simulink model "stream_mdbrt_backup5"  (R2023b)
settings: Solver=VariableStepAuto  StartTime=0.0  StopTime=(48)/fs  RelTol=1e-3
PreLoadFcn:
  | clear all;
  | 
  | fs = 100e6;
PostLoadFcn:
  | ratio = 1/6;
  | set(0,'units','pixels');
  | pixels = get(0,'screensize');
  | point1 = round(pixels(3)*ratio);
  | point2 = round(pixels(4)*ratio);
  | point3 = pixels(3)-round(pixels(3)*ratio);
  | point4 = pixels(4)-round(pixels(4)*ratio);
  | h = get_param(gcs,'handle');
  | set_param(h,'location',[point1 point2 point3 point4]);
  | pause(0.2);
  | set_param(h,'Zoomfactor','fit to view');
  | 
  | clear ratio pixels point1 point2 point3 point4 h
  | 
  | % https://uk.mathworks.com/matlabcentral/answers/358413-open-simulink-model-with-set-window-size-and-position
undefined symbols (not defined in the file): AXI4, bits, bitsheight, bitsiter, bitswidth, Lite, xc7z020clg400
libraries: hdlBasic x527, vmcUtilities x1
(part 5 of 5)

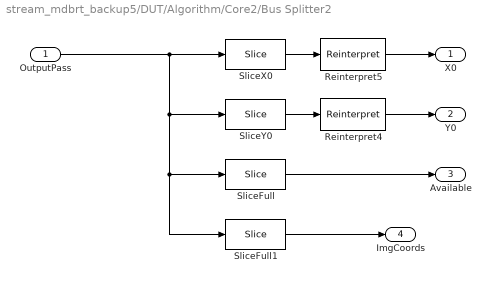
== system stream_mdbrt_backup5/DUT/Algorithm/Core2/Bus Splitter2 ==
  OutputPass : Inport
  Reinterpret4 : hdlBasic/Reinterpret  force_arith_type=on  arith_type="Signed  (2's comp)"  force_bin_pt=on  bin_pt=binpoint  XmcBlockStatus=1  maskContainerNames=group1  block_type=reinterpret  block_config=sysgen:Reinterpret_config
  Reinterpret5 : hdlBasic/Reinterpret  force_arith_type=on  arith_type="Signed  (2's comp)"  force_bin_pt=on  bin_pt=binpoint  XmcBlockStatus=1  maskContainerNames=group1  block_type=reinterpret  block_config=sysgen:Reinterpret_config
  SliceFull : hdlBasic/Slice  nbits=1  boolean_output=on  mode=Upper Bit Location + Width  bit1=0  base1=MSB of Input  bit0=0  base0=LSB of Input  XmcBlockStatus=1  maskContainerNames=group1  block_type=slice  block_config=sysgen:Slice_config
  SliceFull1 : hdlBasic/Slice  nbits=bitswidth+bitsheight  boolean_output=off  mode=Lower Bit Location + Width  bit1=0  base1=MSB of Input  bit0=0  base0=LSB of Input  XmcBlockStatus=1  maskContainerNames=group1  block_type=slice  block_config=sysgen:Slice_config
  SliceX0 : hdlBasic/Slice  nbits=bits  boolean_output=off  mode=Upper Bit Location + Width  bit1=-1-bits  base1=MSB of Input  bit0=0  base0=LSB of Input  XmcBlockStatus=1  maskContainerNames=group1  block_type=slice  block_config=sysgen:Slice_config
  SliceY0 : hdlBasic/Slice  nbits=bits  boolean_output=off  mode=Upper Bit Location + Width  bit1=-1  base1=MSB of Input  bit0=0  base0=LSB of Input  XmcBlockStatus=1  maskContainerNames=group1  block_type=slice  block_config=sysgen:Slice_config
  X0 : Outport
  Y0 : Outport  Port=2
  Available : Outport  Port=3
  ImgCoords : Outport  Port=4
  wires:
  Reinterpret5/1 -> X0/1
  SliceFull/1 -> Available/1
  Reinterpret4/1 -> Y0/1
  SliceX0/1 -> Reinterpret5/1
  SliceY0/1 -> Reinterpret4/1
  SliceFull1/1 -> ImgCoords/1
  OutputPass/1 -> SliceX0/1, SliceY0/1, SliceFull/1, SliceFull1/1

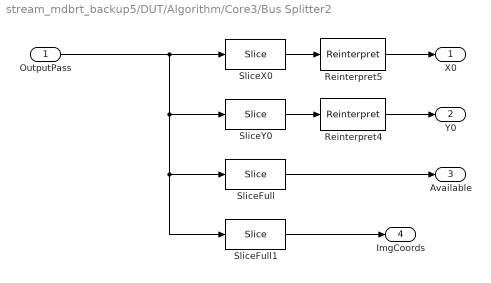
== system stream_mdbrt_backup5/DUT/Algorithm/Core3/Bus Splitter2 ==
  OutputPass : Inport
  Reinterpret4 : hdlBasic/Reinterpret  force_arith_type=on  arith_type="Signed  (2's comp)"  force_bin_pt=on  bin_pt=binpoint  XmcBlockStatus=1  maskContainerNames=group1  block_type=reinterpret  block_config=sysgen:Reinterpret_config
  Reinterpret5 : hdlBasic/Reinterpret  force_arith_type=on  arith_type="Signed  (2's comp)"  force_bin_pt=on  bin_pt=binpoint  XmcBlockStatus=1  maskContainerNames=group1  block_type=reinterpret  block_config=sysgen:Reinterpret_config
  SliceFull : hdlBasic/Slice  nbits=1  boolean_output=on  mode=Upper Bit Location + Width  bit1=0  base1=MSB of Input  bit0=0  base0=LSB of Input  XmcBlockStatus=1  maskContainerNames=group1  block_type=slice  block_config=sysgen:Slice_config
  SliceFull1 : hdlBasic/Slice  nbits=bitswidth+bitsheight  boolean_output=off  mode=Lower Bit Location + Width  bit1=0  base1=MSB of Input  bit0=0  base0=LSB of Input  XmcBlockStatus=1  maskContainerNames=group1  block_type=slice  block_config=sysgen:Slice_config
  SliceX0 : hdlBasic/Slice  nbits=bits  boolean_output=off  mode=Upper Bit Location + Width  bit1=-1-bits  base1=MSB of Input  bit0=0  base0=LSB of Input  XmcBlockStatus=1  maskContainerNames=group1  block_type=slice  block_config=sysgen:Slice_config
  SliceY0 : hdlBasic/Slice  nbits=bits  boolean_output=off  mode=Upper Bit Location + Width  bit1=-1  base1=MSB of Input  bit0=0  base0=LSB of Input  XmcBlockStatus=1  maskContainerNames=group1  block_type=slice  block_config=sysgen:Slice_config
  X0 : Outport
  Y0 : Outport  Port=2
  Available : Outport  Port=3
  ImgCoords : Outport  Port=4
  wires:
  OutputPass/1 -> SliceFull1/1, SliceFull/1, SliceY0/1, SliceX0/1
  SliceFull1/1 -> ImgCoords/1
  SliceY0/1 -> Reinterpret4/1
  SliceX0/1 -> Reinterpret5/1
  Reinterpret4/1 -> Y0/1
  SliceFull/1 -> Available/1
  Reinterpret5/1 -> X0/1

== system stream_mdbrt_backup5/DUT/Algorithm/Core4/Bus Splitter2 ==
  OutputPass : Inport
  Reinterpret4 : hdlBasic/Reinterpret  force_arith_type=on  arith_type="Signed  (2's comp)"  force_bin_pt=on  bin_pt=binpoint  XmcBlockStatus=1  maskContainerNames=group1  block_type=reinterpret  block_config=sysgen:Reinterpret_config
  Reinterpret5 : hdlBasic/Reinterpret  force_arith_type=on  arith_type="Signed  (2's comp)"  force_bin_pt=on  bin_pt=binpoint  XmcBlockStatus=1  maskContainerNames=group1  block_type=reinterpret  block_config=sysgen:Reinterpret_config
  SliceFull : hdlBasic/Slice  nbits=1  boolean_output=on  mode=Upper Bit Location + Width  bit1=0  base1=MSB of Input  bit0=0  base0=LSB of Input  XmcBlockStatus=1  maskContainerNames=group1  block_type=slice  block_config=sysgen:Slice_config
  SliceFull1 : hdlBasic/Slice  nbits=bitswidth+bitsheight  boolean_output=off  mode=Lower Bit Location + Width  bit1=0  base1=MSB of Input  bit0=0  base0=LSB of Input  XmcBlockStatus=1  maskContainerNames=group1  block_type=slice  block_config=sysgen:Slice_config
  SliceX0 : hdlBasic/Slice  nbits=bits  boolean_output=off  mode=Upper Bit Location + Width  bit1=-1-bits  base1=MSB of Input  bit0=0  base0=LSB of Input  XmcBlockStatus=1  maskContainerNames=group1  block_type=slice  block_config=sysgen:Slice_config
  SliceY0 : hdlBasic/Slice  nbits=bits  boolean_output=off  mode=Upper Bit Location + Width  bit1=-1  base1=MSB of Input  bit0=0  base0=LSB of Input  XmcBlockStatus=1  maskContainerNames=group1  block_type=slice  block_config=sysgen:Slice_config
  X0 : Outport
  Y0 : Outport  Port=2
  Available : Outport  Port=3
  ImgCoords : Outport  Port=4
  wires:
  Reinterpret5/1 -> X0/1
  SliceFull/1 -> Available/1
  Reinterpret4/1 -> Y0/1
  SliceX0/1 -> Reinterpret5/1
  SliceY0/1 -> Reinterpret4/1
  SliceFull1/1 -> ImgCoords/1
  OutputPass/1 -> SliceX0/1, SliceY0/1, SliceFull/1, SliceFull1/1

== system stream_mdbrt_backup5/DUT/Algorithm/Core5/Bus Splitter2 ==
  OutputPass : Inport
  Reinterpret4 : hdlBasic/Reinterpret  force_arith_type=on  arith_type="Signed  (2's comp)"  force_bin_pt=on  bin_pt=binpoint  XmcBlockStatus=1  maskContainerNames=group1  block_type=reinterpret  block_config=sysgen:Reinterpret_config
  Reinterpret5 : hdlBasic/Reinterpret  force_arith_type=on  arith_type="Signed  (2's comp)"  force_bin_pt=on  bin_pt=binpoint  XmcBlockStatus=1  maskContainerNames=group1  block_type=reinterpret  block_config=sysgen:Reinterpret_config
  SliceFull : hdlBasic/Slice  nbits=1  boolean_output=on  mode=Upper Bit Location + Width  bit1=0  base1=MSB of Input  bit0=0  base0=LSB of Input  XmcBlockStatus=1  maskContainerNames=group1  block_type=slice  block_config=sysgen:Slice_config
  SliceFull1 : hdlBasic/Slice  nbits=bitswidth+bitsheight  boolean_output=off  mode=Lower Bit Location + Width  bit1=0  base1=MSB of Input  bit0=0  base0=LSB of Input  XmcBlockStatus=1  maskContainerNames=group1  block_type=slice  block_config=sysgen:Slice_config
  SliceX0 : hdlBasic/Slice  nbits=bits  boolean_output=off  mode=Upper Bit Location + Width  bit1=-1-bits  base1=MSB of Input  bit0=0  base0=LSB of Input  XmcBlockStatus=1  maskContainerNames=group1  block_type=slice  block_config=sysgen:Slice_config
  SliceY0 : hdlBasic/Slice  nbits=bits  boolean_output=off  mode=Upper Bit Location + Width  bit1=-1  base1=MSB of Input  bit0=0  base0=LSB of Input  XmcBlockStatus=1  maskContainerNames=group1  block_type=slice  block_config=sysgen:Slice_config
  X0 : Outport
  Y0 : Outport  Port=2
  Available : Outport  Port=3
  ImgCoords : Outport  Port=4
  wires:
  OutputPass/1 -> SliceFull1/1, SliceFull/1, SliceY0/1, SliceX0/1
  SliceFull1/1 -> ImgCoords/1
  SliceY0/1 -> Reinterpret4/1
  SliceX0/1 -> Reinterpret5/1
  Reinterpret4/1 -> Y0/1
  SliceFull/1 -> Available/1
  Reinterpret5/1 -> X0/1

== system stream_mdbrt_backup5/DUT/Algorithm/Core6/Bus Splitter2 ==
  OutputPass : Inport
  Reinterpret4 : hdlBasic/Reinterpret  force_arith_type=on  arith_type="Signed  (2's comp)"  force_bin_pt=on  bin_pt=binpoint  XmcBlockStatus=1  maskContainerNames=group1  block_type=reinterpret  block_config=sysgen:Reinterpret_config
  Reinterpret5 : hdlBasic/Reinterpret  force_arith_type=on  arith_type="Signed  (2's comp)"  force_bin_pt=on  bin_pt=binpoint  XmcBlockStatus=1  maskContainerNames=group1  block_type=reinterpret  block_config=sysgen:Reinterpret_config
  SliceFull : hdlBasic/Slice  nbits=1  boolean_output=on  mode=Upper Bit Location + Width  bit1=0  base1=MSB of Input  bit0=0  base0=LSB of Input  XmcBlockStatus=1  maskContainerNames=group1  block_type=slice  block_config=sysgen:Slice_config
  SliceFull1 : hdlBasic/Slice  nbits=bitswidth+bitsheight  boolean_output=off  mode=Lower Bit Location + Width  bit1=0  base1=MSB of Input  bit0=0  base0=LSB of Input  XmcBlockStatus=1  maskContainerNames=group1  block_type=slice  block_config=sysgen:Slice_config
  SliceX0 : hdlBasic/Slice  nbits=bits  boolean_output=off  mode=Upper Bit Location + Width  bit1=-1-bits  base1=MSB of Input  bit0=0  base0=LSB of Input  XmcBlockStatus=1  maskContainerNames=group1  block_type=slice  block_config=sysgen:Slice_config
  SliceY0 : hdlBasic/Slice  nbits=bits  boolean_output=off  mode=Upper Bit Location + Width  bit1=-1  base1=MSB of Input  bit0=0  base0=LSB of Input  XmcBlockStatus=1  maskContainerNames=group1  block_type=slice  block_config=sysgen:Slice_config
  X0 : Outport
  Y0 : Outport  Port=2
  Available : Outport  Port=3
  ImgCoords : Outport  Port=4
  wires:
  Reinterpret5/1 -> X0/1
  SliceFull/1 -> Available/1
  Reinterpret4/1 -> Y0/1
  SliceX0/1 -> Reinterpret5/1
  SliceY0/1 -> Reinterpret4/1
  SliceFull1/1 -> ImgCoords/1
  OutputPass/1 -> SliceX0/1, SliceY0/1, SliceFull/1, SliceFull1/1
